simulink model "packetLoss"  (R2017a)
settings: Solver=VariableStepAuto  StartTime=0.0  StopTime=simulationTime  RelTol=1e-3
values from neighbouring files (symbols this model uses):
  Acont = [0 1;0 0]    [delayRMPC.m]    (also in runPL.m; runRMPC.m; simul1.mat = [0  1; 0  0]; simul10.mat = [0  1; 0  0])
  Ades = [rell1,ALB;rell1,AUB;rell2,ADeltaLB,rell3;rell2,rell3,ADeltaLB;rell2,ADeltaUB,rell3;rell2,rell3,ADeltaUB]    [defRestricciones.m]    (also in simul1.mat = [0 0 0 0 0 0 0 0 0 0 0 0 ... (1080 elements, 36x30)]; simul10.mat = [0 0 0 0 0 0 0 0 0 0 0 0 ... (1080 elements, 36x30)]; simul11.mat = [0 0 0 0 0 0 0 0 0 0 0 0 ... (1080 elements, 36x30)]; simul12.mat = [0 0 0 0 0 0 0 0 0 0 0 0 ... (1080 elements, 36x30)])
  Bcont = [0;1]    [delayRMPC.m]    (also in runPL.m; runRMPC.m; simul1.mat = [0 1]; simul10.mat = [0 1])
  bdes = [bLB;bUB;bDeltaLB;bDeltaUB]    [defRestricciones.m]    (also in simul1.mat = [1.5 1.5 1.5 1.5 1.5 1.5 1.5 1.5 1.5 1.5 1 1 ... (36 element; simul10.mat = [1.5 1.5 1.5 1.5 1.5 1.5 1.5 1.5 1.5 1.5 1 1 ... (36 element; simul11.mat = [1.5 1.5 1.5 1.5 1.5 1.5 1.5 1.5 1.5 1.5 1 1 ... (36 element; simul12.mat = [1.5 1.5 1.5 1.5 1.5 1.5 1.5 1.5 1.5 1.5 1 1 ... (36 element)
  Ccont = eye(2)    [delayRMPC.m]    (also in runPL.m; runRMPC.m; simul1.mat = [1  0; 0  1]; simul10.mat = [1  0; 0  1])
  d = 2    [delayRMPC.m]    (also in runPL.m; runRMPC.m; simul1.mat; simul10.mat)
  Dcont = [0;0]    [delayRMPC.m]    (also in runPL.m; runRMPC.m; simul1.mat = [0 0]; simul10.mat = [0 0])
  Ldes = input('Valor de spacing deseado (m): ')    [delayRMPC.m]    (also in runPL.m; runRMPC.m; simul1.mat = 2; simul10.mat = 2)
  meanError = -0.0091    [delayRMPC.m]    (also in runPL.m; runRMPC.m; simul1.mat = 0.0164; simul10.mat = 0.0164)
  MError =     [simul1.mat]    (also in simul10.mat; simul11.mat; simul12.mat; simul13.mat)
  nPasos = (length(bdes)+4)/8    [comprimirRestricciones.m]    (also in delayRMPC.m = input('Numero de pasos prediccion: '); runPL.m = input('Numero de pasos prediccion: '); runRMPC.m = input('Numero de pasos prediccion: '); simul1.mat = 5)
  PER = input('PER:')    [runPL.m]    (also in simul10.mat = 0.01; simul11.mat = 0.1; simul12.mat = 0.2; simul13.mat = 0.3)
  transmissionDelay = input('Delay (ms)')/1000    [delayRMPC.m]    (also in runPL.m; simul1.mat = 0; simul10.mat = 0.0001; simul11.mat = 0.0001)
  ts = input('Tiempo de muestreo (s): ')    [delayRMPC.m]    (also in runPL.m; runRMPC.m; simul1.mat = 0.4; simul10.mat = 0.5)
  v0Bici1 = 1    [delayRMPC.m]    (also in runPL.m; runRMPC.m; simul1.mat; simul10.mat)
  v0Bici2 = 1    [delayRMPC.m]    (also in runPL.m; runRMPC.m; simul1.mat; simul10.mat)
  v0Bici3 = 1    [delayRMPC.m]    (also in runPL.m; runRMPC.m; simul1.mat; simul10.mat)
  v0Bici4 = 1    [delayRMPC.m]    (also in runPL.m; simul1.mat; simul10.mat; simul11.mat)
  v0Leader = input('Velocidad lider (m/s)(2.7,4.16,5)')    [delayRMPC.m]    (also in runPL.m; runRMPC.m; simul1.mat = 2.7; simul10.mat = 2.7)
  varError = varError^2    (= 0.15800625)    [delayRMPC.m]    (also in runPL.m; runRMPC.m; simul1.mat = 0.14661241; simul10.mat = 0.14661241)
  x0Bici1 = -10    [delayRMPC.m]    (also in runPL.m; runRMPC.m; simul1.mat; simul10.mat)
  x0Bici2 = -20    [delayRMPC.m]    (also in runPL.m; runRMPC.m; simul1.mat; simul10.mat)
  x0Bici3 = -30    [delayRMPC.m]    (also in runPL.m; runRMPC.m; simul1.mat; simul10.mat)
  x0Bici4 = -40    [delayRMPC.m]    (also in runPL.m; simul1.mat; simul10.mat; simul11.mat)
  x0Leader = 0    [delayRMPC.m]    (also in runPL.m; runRMPC.m; simul1.mat; simul10.mat)
undefined symbols (not defined in the file or in its folder): solveRMPC
settings Model: Creator=tlara  LastModifiedBy=tlara

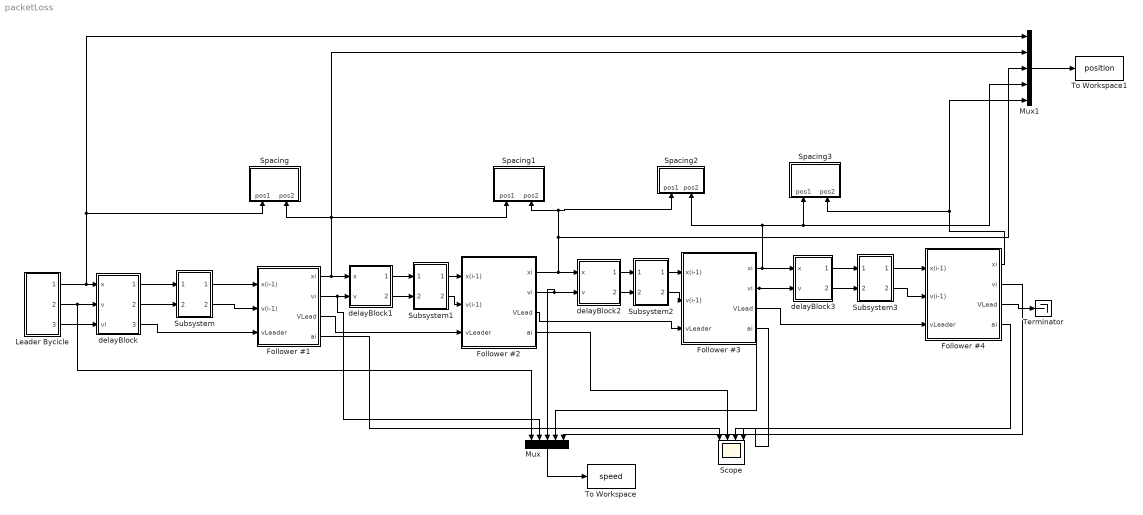
== system packetLoss ==
  "Follower #1 " : Subsystem
  Follower #2 : Subsystem
  Follower #3 : Subsystem
  Follower #4 : Subsystem
  "Leader Bycicle " : Subsystem
  Mux : Mux  Inputs=5
  Mux1 : Mux  Inputs=5
  Scope : Scope  NumInputPorts=4
  Spacing : Subsystem
  Spacing1 : Subsystem
  Spacing2 : Subsystem
  Spacing3 : Subsystem
  Subsystem : Subsystem
  Subsystem1 : Subsystem
  Subsystem2 : Subsystem
  Subsystem3 : Subsystem
  Terminator : Terminator
  To Workspace : ToWorkspace  VariableName=speed  SaveFormat=Timeseries  SampleTime=-1
  To Workspace1 : ToWorkspace  VariableName=position  SaveFormat=Timeseries  SampleTime=-1
  delayBlock : Subsystem
  delayBlock1 : Subsystem
  delayBlock2 : Subsystem
  delayBlock3 : Subsystem
  wires:
  Mux/1 -> To Workspace/1
  Follower #4/3(VLead) -> Terminator/1
  Mux1/1 -> To Workspace1/1
  "Leader Bycicle "/1(Position) -> Spacing/1(pos1), Mux1/1, delayBlock/1(x)
  "Leader Bycicle "/2(Speed) -> Mux/1, delayBlock/2(v)
  "Leader Bycicle "/3(lSpeed) -> delayBlock/3(vl)
  delayBlock/2(delayV) -> Subsystem/2("Vin ")
  delayBlock/1(delayX) -> Subsystem/1(Xin)
  Subsystem/1(XOut) -> "Follower #1 "/1(x(i-1))
  Subsystem/2(VOut) -> "Follower #1 "/2(v(i-1))
  delayBlock/3(delayVl) -> "Follower #1 "/3(vLeader)
  "Follower #1 "/1(xi) -> Spacing/2(pos2), Spacing1/1(pos1), Mux1/2, delayBlock1/1(x)
  "Follower #1 "/2(vi) -> Mux/2, delayBlock1/2(v)
  Follower #2/1(xi) -> delayBlock2/1(x), Spacing2/1(pos1), Spacing1/2(pos2), Mux1/3
  "Follower #1 "/3(VLead) -> Follower #2/3(vLeader)
  Follower #2/3(VLead) -> Follower #3/3(vLeader)
  "Follower #1 "/4(ai) -> Scope/1
  Follower #2/4(ai) -> Scope/2
  Follower #3/4(ai) -> Scope/3
  Follower #3/2(vi) -> Mux/4, delayBlock3/2(v)
  Follower #3/1(xi) -> Spacing2/2(pos2), Spacing3/1(pos1), Mux1/4, delayBlock3/1(x)
  Follower #4/4(ai) -> Scope/4
  Follower #4/2(vi) -> Mux/5
  Follower #4/1(xi) -> Spacing3/2(pos2), Mux1/5
  Subsystem1/1(XOut) -> Follower #2/1(x(i-1))
  delayBlock1/1(delayX) -> Subsystem1/1(Xin)
  delayBlock1/2(delayV) -> Subsystem1/2("Vin ")
  Subsystem1/2(VOut) -> Follower #2/2(v(i-1))
  Follower #2/2(vi) -> Mux/3, delayBlock2/2(v)
  delayBlock2/1(delayX) -> Subsystem2/1(Xin)
  delayBlock2/2(delayV) -> Subsystem2/2("Vin ")
  Subsystem2/1(XOut) -> Follower #3/1(x(i-1))
  Subsystem2/2(VOut) -> Follower #3/2(v(i-1))
  Follower #3/3(VLead) -> Follower #4/3(vLeader)
  delayBlock3/2(delayV) -> Subsystem3/2("Vin ")
  delayBlock3/1(delayX) -> Subsystem3/1(Xin)
  Subsystem3/1(XOut) -> Follower #4/1(x(i-1))
  Subsystem3/2(VOut) -> Follower #4/2(v(i-1))

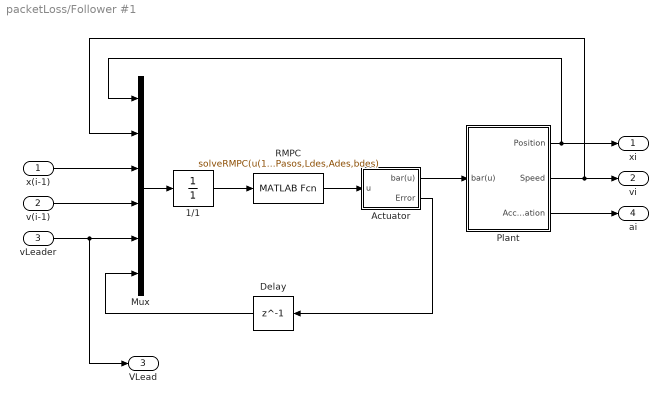
== system packetLoss/Follower #1  ==
  x(i-1) : Inport
  v(i-1) : Inport  Port=2
  vLeader : Inport  Port=3
  "1/1 " : DiscreteTransferFcn  Denominator=[1]  SampleTime=ts
  Actuator : Subsystem
  Delay : Delay  DelayLength=1  InitialCondition=0  SampleTime=ts
  Mux : Mux  Inputs=6
  Plant : Subsystem
  RMPC : MATLABFcn  MATLABFcn=solveRMPC(u(1),u(2),u(3),u(4),u(5),u(6),MError,nPasos,Ldes,Ades,bdes)  OutputDimensions=1  OutputSignalType=real
  xi : Outport
  vi : Outport  Port=2
  VLead : Outport  Port=3
  ai : Outport  Port=4
  wires:
  vLeader/1 -> VLead/1, Mux/5
  v(i-1)/1 -> Mux/4
  x(i-1)/1 -> Mux/3
  Mux/1 -> "1/1 "/1
  "1/1 "/1 -> RMPC/1
  RMPC/1 -> Actuator/1(u)
  Actuator/1(bar(u)) -> Plant/1(bar(u))
  Plant/1(Position) -> Mux/1, xi/1
  Plant/2("Speed ") -> Mux/2, vi/1
  Plant/3(Acceleration) -> ai/1
  Actuator/2(Error) -> Delay/1
  Delay/1 -> Mux/6

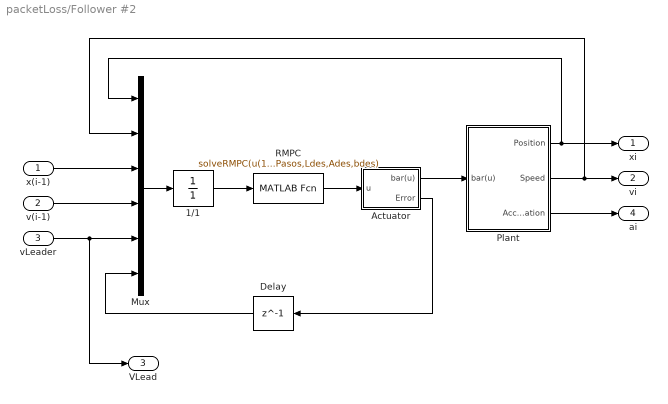
== system packetLoss/Follower #2 ==
  x(i-1) : Inport
  v(i-1) : Inport  Port=2
  vLeader : Inport  Port=3
  "1/1 " : DiscreteTransferFcn  Denominator=[1]  SampleTime=ts
  Actuator : Subsystem
  Delay : Delay  DelayLength=1  InitialCondition=0  SampleTime=ts
  Mux : Mux  Inputs=6
  Plant : Subsystem
  RMPC : MATLABFcn  MATLABFcn=solveRMPC(u(1),u(2),u(3),u(4),u(5),u(6),MError,nPasos,Ldes,Ades,bdes)  OutputDimensions=1  OutputSignalType=real
  xi : Outport
  vi : Outport  Port=2
  VLead : Outport  Port=3
  ai : Outport  Port=4
  wires:
  vLeader/1 -> VLead/1, Mux/5
  v(i-1)/1 -> Mux/4
  x(i-1)/1 -> Mux/3
  Mux/1 -> "1/1 "/1
  "1/1 "/1 -> RMPC/1
  RMPC/1 -> Actuator/1(u)
  Actuator/1(bar(u)) -> Plant/1(bar(u))
  Plant/1(Position) -> Mux/1, xi/1
  Plant/2("Speed ") -> Mux/2, vi/1
  Plant/3(Acceleration) -> ai/1
  Actuator/2(Error) -> Delay/1
  Delay/1 -> Mux/6

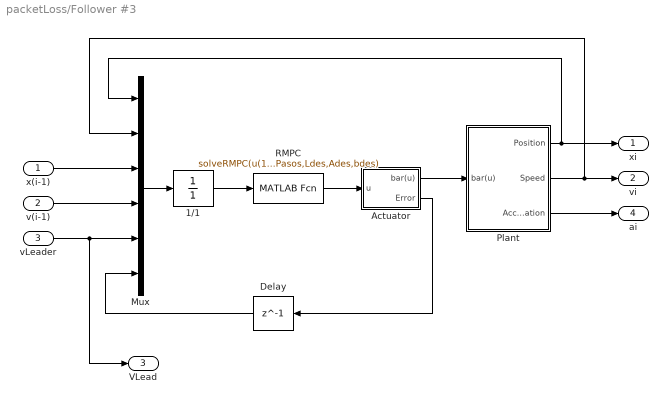
== system packetLoss/Follower #3 ==
  x(i-1) : Inport
  v(i-1) : Inport  Port=2
  vLeader : Inport  Port=3
  "1/1 " : DiscreteTransferFcn  Denominator=[1]  SampleTime=ts
  Actuator : Subsystem
  Delay : Delay  DelayLength=1  InitialCondition=0  SampleTime=ts
  Mux : Mux  Inputs=6
  Plant : Subsystem
  RMPC : MATLABFcn  MATLABFcn=solveRMPC(u(1),u(2),u(3),u(4),u(5),u(6),MError,nPasos,Ldes,Ades,bdes)  OutputDimensions=1  OutputSignalType=real
  xi : Outport
  vi : Outport  Port=2
  VLead : Outport  Port=3
  ai : Outport  Port=4
  wires:
  vLeader/1 -> VLead/1, Mux/5
  v(i-1)/1 -> Mux/4
  x(i-1)/1 -> Mux/3
  Mux/1 -> "1/1 "/1
  "1/1 "/1 -> RMPC/1
  RMPC/1 -> Actuator/1(u)
  Actuator/1(bar(u)) -> Plant/1(bar(u))
  Plant/1(Position) -> Mux/1, xi/1
  Plant/2("Speed ") -> Mux/2, vi/1
  Plant/3(Acceleration) -> ai/1
  Actuator/2(Error) -> Delay/1
  Delay/1 -> Mux/6

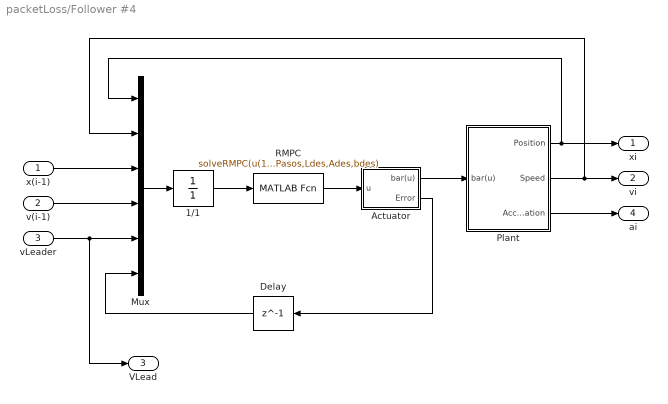
== system packetLoss/Follower #4 ==
  x(i-1) : Inport
  v(i-1) : Inport  Port=2
  vLeader : Inport  Port=3
  "1/1 " : DiscreteTransferFcn  Denominator=[1]  SampleTime=ts
  Actuator : Subsystem
  Delay : Delay  DelayLength=1  InitialCondition=0  SampleTime=ts
  Mux : Mux  Inputs=6
  Plant : Subsystem
  RMPC : MATLABFcn  MATLABFcn=solveRMPC(u(1),u(2),u(3),u(4),u(5),u(6),MError,nPasos,Ldes,Ades,bdes)  OutputDimensions=1  OutputSignalType=real
  xi : Outport
  vi : Outport  Port=2
  VLead : Outport  Port=3
  ai : Outport  Port=4
  wires:
  vLeader/1 -> VLead/1, Mux/5
  v(i-1)/1 -> Mux/4
  x(i-1)/1 -> Mux/3
  Mux/1 -> "1/1 "/1
  "1/1 "/1 -> RMPC/1
  RMPC/1 -> Actuator/1(u)
  Actuator/1(bar(u)) -> Plant/1(bar(u))
  Plant/1(Position) -> Mux/1, xi/1
  Plant/2("Speed ") -> Mux/2, vi/1
  Plant/3(Acceleration) -> ai/1
  Actuator/2(Error) -> Delay/1
  Delay/1 -> Mux/6

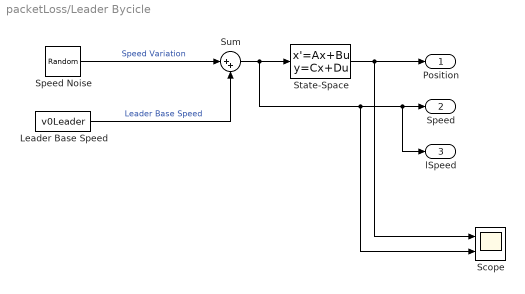
== system packetLoss/Leader Bycicle  ==
  "Leader Base Speed " : Constant  Value=v0Leader
  Scope : Scope  NumInputPorts=2
  Speed Noise : RandomNumber  Variance=0.02  SampleTime=ts
  State-Space : StateSpace  A=[0]  B=[1]  C=[1]  D=[0]  X0=[x0Leader]  ContinuousStateAttributes='position'
  Sum : Sum  Inputs=|++
  Position : Outport
  Speed : Outport  Port=2
  lSpeed : Outport  Port=3
  wires:
  "Leader Base Speed "/1 -> Sum/2  "Leader Base Speed"
  Speed Noise/1 -> Sum/1  "Speed Variation"
  State-Space/1 -> Position/1, Scope/1
  Sum/1 -> State-Space/1, lSpeed/1, Speed/1, Scope/2

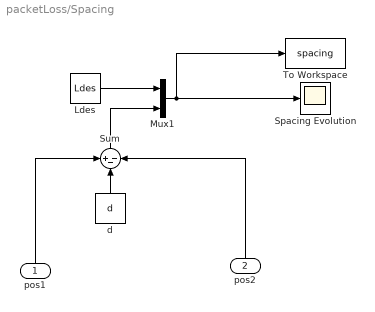
== system packetLoss/Spacing ==
  pos1 : Inport
  pos2 : Inport  Port=2
  Ldes : Constant  Value=Ldes
  Mux1 : Mux  Inputs=2
  Spacing Evolution : Scope
  Sum : Sum  Inputs=+--
  To Workspace : ToWorkspace  VariableName=spacing  SaveFormat=Timeseries  SampleTime=-1
  "d " : Constant  Value=d
  wires:
  Ldes/1 -> Mux1/1
  "d "/1 -> Sum/2
  pos2/1 -> Sum/3
  pos1/1 -> Sum/1
  Sum/1 -> Mux1/2
  Mux1/1 -> To Workspace/1, Spacing Evolution/1

== system packetLoss/Spacing1 ==
  pos1 : Inport
  pos2 : Inport  Port=2
  Ldes : Constant  Value=Ldes
  Mux1 : Mux  Inputs=2
  Spacing Evolution : Scope
  Sum : Sum  Inputs=+--
  To Workspace : ToWorkspace  VariableName=spacing2  SaveFormat=Timeseries  SampleTime=-1
  "d " : Constant  Value=d
  wires:
  Ldes/1 -> Mux1/1
  "d "/1 -> Sum/2
  pos2/1 -> Sum/3
  pos1/1 -> Sum/1
  Sum/1 -> Mux1/2
  Mux1/1 -> To Workspace/1, Spacing Evolution/1

== system packetLoss/Spacing2 ==
  pos1 : Inport
  pos2 : Inport  Port=2
  Ldes : Constant  Value=Ldes
  Mux1 : Mux  Inputs=2
  Spacing Evolution : Scope
  Sum : Sum  Inputs=+--
  To Workspace : ToWorkspace  VariableName=spacing3  SaveFormat=Timeseries  SampleTime=-1
  "d " : Constant  Value=d
  wires:
  Ldes/1 -> Mux1/1
  "d "/1 -> Sum/2
  pos2/1 -> Sum/3
  pos1/1 -> Sum/1
  Sum/1 -> Mux1/2
  Mux1/1 -> To Workspace/1, Spacing Evolution/1

== system packetLoss/Spacing3 ==
  pos1 : Inport
  pos2 : Inport  Port=2
  Ldes : Constant  Value=Ldes
  Mux1 : Mux  Inputs=2
  Spacing Evolution : Scope
  Sum : Sum  Inputs=+--
  To Workspace : ToWorkspace  VariableName=spacing4  SaveFormat=Timeseries  SampleTime=-1
  "d " : Constant  Value=d
  wires:
  Ldes/1 -> Mux1/1
  "d "/1 -> Sum/2
  pos2/1 -> Sum/3
  pos1/1 -> Sum/1
  Sum/1 -> Mux1/2
  Mux1/1 -> To Workspace/1, Spacing Evolution/1

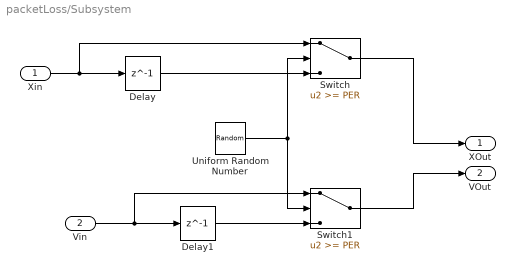
== system packetLoss/Subsystem ==
  Xin : Inport
  "Vin " : Inport  Port=2
  Delay : Delay  DelayLength=1  SampleTime=ts
  Delay1 : Delay  DelayLength=1  SampleTime=ts
  Switch : Switch  Threshold=PER
  Switch1 : Switch  Threshold=PER
  Uniform Random Number : UniformRandomNumber  Seed=4  SampleTime=0.1
  XOut : Outport
  VOut : Outport  Port=2
  wires:
  "Vin "/1 -> Switch1/1, Delay1/1
  Xin/1 -> Switch/1, Delay/1
  Switch1/1 -> VOut/1
  Switch/1 -> XOut/1
  Delay1/1 -> Switch1/3
  Uniform Random Number/1 -> Switch/2, Switch1/2
  Delay/1 -> Switch/3

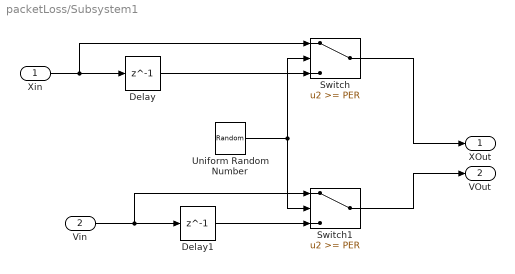
== system packetLoss/Subsystem1 ==
  Xin : Inport
  "Vin " : Inport  Port=2
  Delay : Delay  DelayLength=1  SampleTime=ts
  Delay1 : Delay  DelayLength=1  SampleTime=ts
  Switch : Switch  Threshold=PER
  Switch1 : Switch  Threshold=PER
  Uniform Random Number : UniformRandomNumber  Seed=20  SampleTime=0.1
  XOut : Outport
  VOut : Outport  Port=2
  wires:
  "Vin "/1 -> Switch1/1, Delay1/1
  Xin/1 -> Switch/1, Delay/1
  Switch1/1 -> VOut/1
  Switch/1 -> XOut/1
  Delay1/1 -> Switch1/3
  Uniform Random Number/1 -> Switch/2, Switch1/2
  Delay/1 -> Switch/3

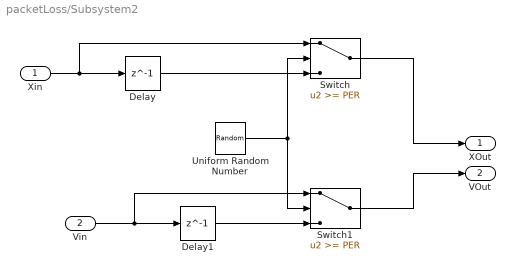
== system packetLoss/Subsystem2 ==
  Xin : Inport
  "Vin " : Inport  Port=2
  Delay : Delay  DelayLength=1  SampleTime=ts
  Delay1 : Delay  DelayLength=1  SampleTime=ts
  Switch : Switch  Threshold=PER
  Switch1 : Switch  Threshold=PER
  Uniform Random Number : UniformRandomNumber  Seed=13  SampleTime=0.1
  XOut : Outport
  VOut : Outport  Port=2
  wires:
  "Vin "/1 -> Switch1/1, Delay1/1
  Xin/1 -> Switch/1, Delay/1
  Switch1/1 -> VOut/1
  Switch/1 -> XOut/1
  Delay1/1 -> Switch1/3
  Uniform Random Number/1 -> Switch/2, Switch1/2
  Delay/1 -> Switch/3

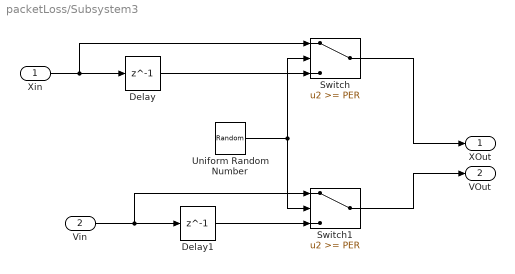
== system packetLoss/Subsystem3 ==
  Xin : Inport
  "Vin " : Inport  Port=2
  Delay : Delay  DelayLength=1  SampleTime=ts
  Delay1 : Delay  DelayLength=1  SampleTime=ts
  Switch : Switch  Threshold=PER
  Switch1 : Switch  Threshold=PER
  Uniform Random Number : UniformRandomNumber  Minimum=0  Seed=7  SampleTime=0.1
  XOut : Outport
  VOut : Outport  Port=2
  wires:
  "Vin "/1 -> Switch1/1, Delay1/1
  Xin/1 -> Switch/1, Delay/1
  Switch1/1 -> VOut/1
  Switch/1 -> XOut/1
  Delay1/1 -> Switch1/3
  Uniform Random Number/1 -> Switch/2, Switch1/2
  Delay/1 -> Switch/3

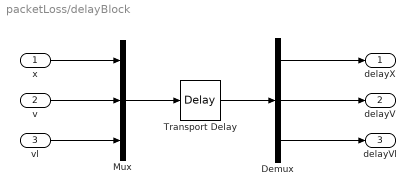
== system packetLoss/delayBlock ==
  x : Inport
  v : Inport  Port=2
  vl : Inport  Port=3
  Demux : Demux  Outputs=3
  Mux : Mux  Inputs=3
  Transport Delay : TransportDelay  DelayTime=transmissionDelay
  delayX : Outport
  delayV : Outport  Port=2
  delayVl : Outport  Port=3
  wires:
  x/1 -> Mux/1
  v/1 -> Mux/2
  vl/1 -> Mux/3
  Mux/1 -> Transport Delay/1
  Transport Delay/1 -> Demux/1
  Demux/1 -> delayX/1
  Demux/2 -> delayV/1
  Demux/3 -> delayVl/1

== system packetLoss/delayBlock1 ==
  x : Inport
  v : Inport  Port=2
  Demux : Demux  Outputs=2
  Mux : Mux  Inputs=2
  Transport Delay : TransportDelay  DelayTime=transmissionDelay
  delayX : Outport
  delayV : Outport  Port=2
  wires:
  x/1 -> Mux/1
  v/1 -> Mux/2
  Mux/1 -> Transport Delay/1
  Transport Delay/1 -> Demux/1
  Demux/1 -> delayX/1
  Demux/2 -> delayV/1

== system packetLoss/delayBlock2 ==
  x : Inport
  v : Inport  Port=2
  Demux : Demux  Outputs=2
  Mux : Mux  Inputs=2
  Transport Delay : TransportDelay  DelayTime=transmissionDelay
  delayX : Outport
  delayV : Outport  Port=2
  wires:
  x/1 -> Mux/1
  v/1 -> Mux/2
  Mux/1 -> Transport Delay/1
  Transport Delay/1 -> Demux/1
  Demux/1 -> delayX/1
  Demux/2 -> delayV/1

== system packetLoss/delayBlock3 ==
  x : Inport
  v : Inport  Port=2
  Demux : Demux  Outputs=2
  Mux : Mux  Inputs=2
  Transport Delay : TransportDelay  DelayTime=transmissionDelay
  delayX : Outport
  delayV : Outport  Port=2
  wires:
  x/1 -> Mux/1
  v/1 -> Mux/2
  Mux/1 -> Transport Delay/1
  Transport Delay/1 -> Demux/1
  Demux/1 -> delayX/1
  Demux/2 -> delayV/1

== system packetLoss/Follower #1 /Actuator ==
  u : Inport
  Actuator Noise : RandomNumber  Mean=meanError  Variance=varError  SampleTime=ts
  Sum : Sum  Inputs=|++
  bar(u) : Outport
  Error : Outport  Port=2
  wires:
  Sum/1 -> bar(u)/1
  u/1 -> Sum/1
  Actuator Noise/1 -> Sum/2, Error/1

== system packetLoss/Follower #1 /Plant ==
  bar(u) : Inport
  Demux : Demux  Outputs=2
  "System (Bicycle) " : StateSpace  A=Acont  B=Bcont  C=Ccont  D=Dcont  X0=[x0Bici1,v0Bici1]  ContinuousStateAttributes='Position'
  Zero-Order Hold : ZeroOrderHold  SampleTime=ts
  Position : Outport
  "Speed " : Outport  Port=2
  Acceleration : Outport  Port=3
  wires:
  bar(u)/1 -> Zero-Order Hold/1
  Zero-Order Hold/1 -> Acceleration/1, "System (Bicycle) "/1
  Demux/1 -> Position/1
  "System (Bicycle) "/1 -> Demux/1  "estado"
  Demux/2 -> "Speed "/1

== system packetLoss/Follower #2/Actuator ==
  u : Inport
  Actuator Noise : RandomNumber  Mean=meanError  Variance=varError  SampleTime=ts
  Sum : Sum  Inputs=|++
  bar(u) : Outport
  Error : Outport  Port=2
  wires:
  Sum/1 -> bar(u)/1
  u/1 -> Sum/1
  Actuator Noise/1 -> Sum/2, Error/1

== system packetLoss/Follower #2/Plant ==
  bar(u) : Inport
  Demux : Demux  Outputs=2
  "System (Bicycle) " : StateSpace  A=Acont  B=Bcont  C=Ccont  D=Dcont  X0=[x0Bici2,v0Bici2]  ContinuousStateAttributes='Position'
  Zero-Order Hold : ZeroOrderHold  SampleTime=ts
  Position : Outport
  "Speed " : Outport  Port=2
  Acceleration : Outport  Port=3
  wires:
  bar(u)/1 -> Zero-Order Hold/1
  Zero-Order Hold/1 -> Acceleration/1, "System (Bicycle) "/1
  Demux/1 -> Position/1
  "System (Bicycle) "/1 -> Demux/1  "estado"
  Demux/2 -> "Speed "/1

== system packetLoss/Follower #3/Actuator ==
  u : Inport
  Actuator Noise : RandomNumber  Mean=meanError  Variance=varError  SampleTime=ts
  Sum : Sum  Inputs=|++
  bar(u) : Outport
  Error : Outport  Port=2
  wires:
  Sum/1 -> bar(u)/1
  u/1 -> Sum/1
  Actuator Noise/1 -> Sum/2, Error/1

== system packetLoss/Follower #3/Plant ==
  bar(u) : Inport
  Demux : Demux  Outputs=2
  "System (Bicycle) " : StateSpace  A=Acont  B=Bcont  C=Ccont  D=Dcont  X0=[x0Bici3,v0Bici3]  ContinuousStateAttributes='Position'
  Zero-Order Hold : ZeroOrderHold  SampleTime=ts
  Position : Outport
  "Speed " : Outport  Port=2
  Acceleration : Outport  Port=3
  wires:
  bar(u)/1 -> Zero-Order Hold/1
  Zero-Order Hold/1 -> Acceleration/1, "System (Bicycle) "/1
  Demux/1 -> Position/1
  "System (Bicycle) "/1 -> Demux/1  "estado"
  Demux/2 -> "Speed "/1

== system packetLoss/Follower #4/Actuator ==
  u : Inport
  Actuator Noise : RandomNumber  Mean=meanError  Variance=varError  SampleTime=ts
  Sum : Sum  Inputs=|++
  bar(u) : Outport
  Error : Outport  Port=2
  wires:
  Sum/1 -> bar(u)/1
  u/1 -> Sum/1
  Actuator Noise/1 -> Sum/2, Error/1

== system packetLoss/Follower #4/Plant ==
  bar(u) : Inport
  Demux : Demux  Outputs=2
  "System (Bicycle) " : StateSpace  A=Acont  B=Bcont  C=Ccont  D=Dcont  X0=[x0Bici4,v0Bici4]  ContinuousStateAttributes='Position'
  Zero-Order Hold : ZeroOrderHold  SampleTime=ts
  Position : Outport
  "Speed " : Outport  Port=2
  Acceleration : Outport  Port=3
  wires:
  bar(u)/1 -> Zero-Order Hold/1
  Zero-Order Hold/1 -> Acceleration/1, "System (Bicycle) "/1
  Demux/1 -> Position/1
  "System (Bicycle) "/1 -> Demux/1  "estado"
  Demux/2 -> "Speed "/1
